simulink model "Serial"  (R2020a)
settings: Solver=FixedStepAuto  StartTime=0.0  StopTime=100  FixedStep=Ts  RelTol=1e-3  EnableMultiTasking=on
undefined symbols (not defined in the file or in its folder): Ts
libraries: raspberrypiCommlib x1, simulink x1
settings Model: Creator=hhiastt  LastModifiedBy=hhiastt
settings SolverCC: PositivePriorityOrder=on
settings OptimizationCC: EnhancedBackFolding=on  PassReuseOutputArgsAs=Individual arguments  ZeroExternalMemoryAtStartup=off  ZeroInternalMemoryAtStartup=off  MaxStackSize=64  OptimizeBlockOrder=speed  DifferentSizesBufferReuse=on  OptimizationCustomize=off  EfficientTunableParamExpr=on
settings DebuggingCC: ParameterTunabilityLossMsg=error
settings HardwareCC: ProdBitPerPointer=32  ProdBitPerSizeT=32  ProdBitPerPtrDiffT=32  ProdLargestAtomicInteger=Long  ProdLargestAtomicFloat=Double  ProdWordSize=32  ProdLongLongMode=on  ProdHWDeviceType=ARM Compatible->ARM Cortex
settings RTWCC: SystemTargetFile=ert.tlc  HardwareBoard=Raspberry Pi  TemplateMakefile=ert_default_tmf  Toolchain=GNU GCC Raspberry Pi  BuildConfiguration=Faster Runs
settings CodeAppCC: ForceParamTrailComments=on  IgnoreCustomStorageClasses=off  OperatorAnnotations=on  SimulinkDataObjDesc=on  SFDataObjDesc=on  InsertBlockDesc=on
settings ERTTargetCC: SupportVariableSizeSignals=on

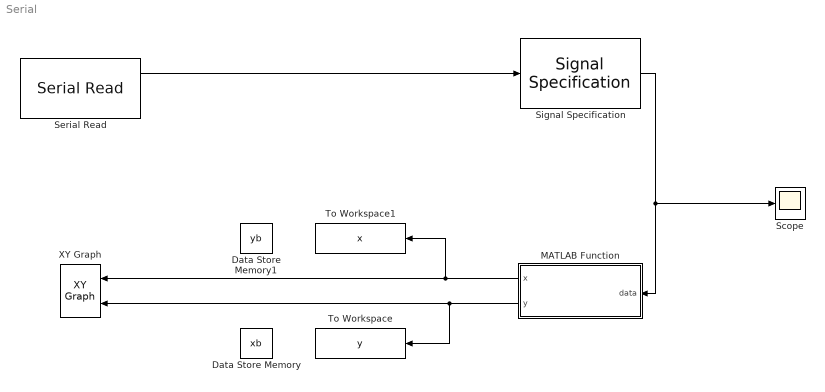
== system Serial ==
  Data Store Memory : DataStoreMemory  DataStoreName=xb  ReadBeforeWriteMsg=warning  WriteAfterWriteMsg=warning  WriteAfterReadMsg=warning  ShowAdditionalParam=off  OutDataTypeStr=double
  Data Store Memory1 : DataStoreMemory  DataStoreName=yb  ReadBeforeWriteMsg=warning  WriteAfterWriteMsg=warning  WriteAfterReadMsg=warning  ShowAdditionalParam=off  OutDataTypeStr=double
  MATLAB Function : MATLAB Function  TreatAsAtomicUnit=on
  Scope : Scope
  Serial Read : raspberrypiCommlib/Serial Read  board=Pi 3 Model B+  SCIModule_=/dev/ttyS0  Baudrate_=19200  Parity=None  StopBits_=1  HardwareFlowControl=None  ByteOrder=LittleEndian  DataLength=10  DataType=uint8  OutputStatus=on  SampleTime=Ts  blockPlatform=RaspberryPi
      settings: SourceProductBaseCode=RASPPI
  Signal Specification : SignalSpecification  OutDataTypeStr=uint8  Dimensions=10  SampleTime=Ts
  To Workspace : ToWorkspace  VariableName=y  SampleTime=Ts
      settings: Save2DSignal=2-D array (concatenate along first dimension)
  To Workspace1 : ToWorkspace  VariableName=x  SampleTime=Ts
      settings: Save2DSignal=2-D array (concatenate along first dimension)
  XY Graph : simulink/Sinks/XY Graph  xmin=0  xmax=30  ymin=0  ymax=30  st=Ts
  wires:
  Signal Specification/1 -> Scope/1, MATLAB Function/1(data)
  MATLAB Function/1(x) -> To Workspace1/1, XY Graph/1
  MATLAB Function/2(y) -> To Workspace/1, XY Graph/2
  Serial Read/1 -> Signal Specification/1

== matlab function Serial/MATLAB Function ==
  data: data input; x output; y output; xb data_store_memory; yb data_store_memory
function [x,y] = process_data(data)
global xb
global yb
x=0;y=0;xx=0;yy=0;j=0;data1=zeros(1,4);
data2=zeros(1,4);
for i=1:10
    if(data(i) == 255)
        j=i;
    end
end
if(j <= 6 && j>0)
    data1=data(j+1:j+4);
    data2=cast(data1,'like',zeros(1,4));    
    xx=data2(1)*256+data2(2);
    yy=data2(3)*256+data2(4);
    xx=(xx-floor(floor(xx/128)/2)*128)/2;
    yy=(yy-floor(floor(yy/128)/2)*128)/2;
    x=((xx-20)/470)*22.8;
    y=((yy-7)/490)*30.4;
    xb=x;
    yb=y;
else
    x=xb;
    y=yb;
end
end
